simulink model "Simulacao_Exemplo_01"  (R2020a)
settings: Solver=ode45  StartTime=0.0  StopTime=240  FixedStep=0.1  MaxStep=5e-1  RelTol=1e-3  EnableMultiTasking=on
settings Model: Creator=MeneghettiAir  LastModifiedBy=jhona
settings DataIOCC: LimitDataPoints=on  SaveFormat=Array  ReturnWorkspaceOutputs=off
settings OptimizationCC: LifeSpan=inf
settings DebuggingCC: SolverPrmCheckMsg=warning  SFUnexpectedBacktrackingDiag=warning  SFNoUnconditionalDefaultTransitionDiag=warning  SFExecutionAtInitializationDiag=none  ArithmeticOperatorsInVariantConditions=warning
settings HardwareCC: ProdBitPerPointer=32  ProdBitPerSizeT=32  ProdBitPerPtrDiffT=32  ProdLargestAtomicFloat=None  ProdIntDivRoundTo=Undefined  ProdEndianess=Unspecified  ProdWordSize=32  ProdHWDeviceType=32-bit Generic
settings ModelReferenceCC: PropagateSignalLabelsOutOfModel=off
settings SFSimCC: SimUseLocalCustomCode=off  CustomCodeUndefinedFunction=UseInterfaceOnly
settings RTWCC: RTWUseLocalCustomCode=off
settings CodeAppCC: StateflowObjectComments=on
settings GRTTargetCC: TargetLangStandard=C89/C90 (ANSI)
settings ConfigComp: CovMetricSettings=dw  CovHtmlReporting=on  CovSaveCumulativeToWorkspaceVar=on  CovSaveSingleToWorkspaceVar=on  CovExternalEMLEnable=off  CovSFcnEnable=off

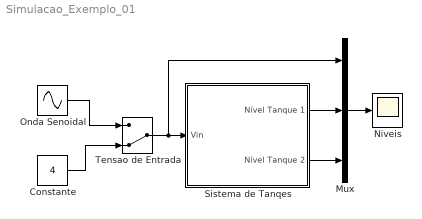
== system Simulacao_Exemplo_01 ==
  Constante : Constant  Value=4  VectorParams1D=off
  Mux : Mux  Inputs=3
  Niveis : Scope
  Onda Senoidal : Sin  Amplitude=2  Bias=2  Frequency=0.2  SampleTime=0
  "Sistema de Tanqes " : Subsystem
  Tensao de Entrada : ManualSwitch  CurrentSetting=0
  wires:
  "Sistema de Tanqes "/1(Nível Tanque 1) -> Mux/2
  "Sistema de Tanqes "/2(Nível Tanque 2) -> Mux/3
  Mux/1 -> Niveis/1
  Tensao de Entrada/1 -> Mux/1, "Sistema de Tanqes "/1(Vin)
  Constante/1 -> Tensao de Entrada/2
  Onda Senoidal/1 -> Tensao de Entrada/1

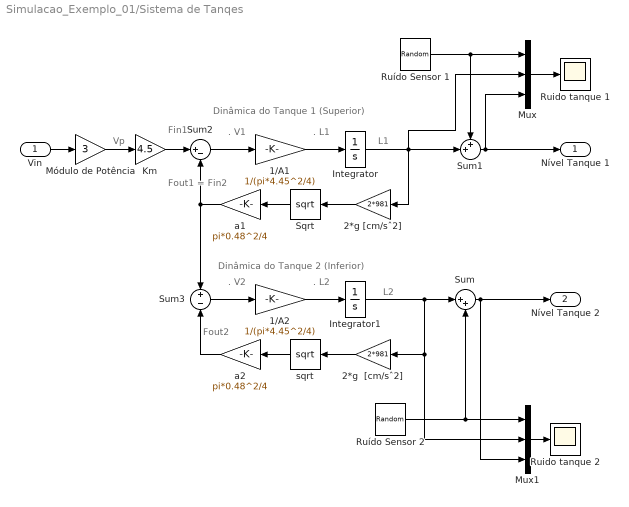
== system Simulacao_Exemplo_01/Sistema de Tanqes  ==
  note: Dinâmica do Tanque 1 (Superior)
  note: L1
  note: Fin1
  note: Fout1
      | =
      | Fin2
  note: .
      | L1
  note: .
      | V1
  note: L2
  note: Fout2
  note: .
      | L2
  note: .
      | V2
  note: Dinâmica do Tanque 2 (Inferior)
  note: Vp
  Vin : Inport
  1/A1 : Gain  Gain=1/(pi*4.45^2/4)
  1/A2 : Gain  Gain=1/(pi*4.45^2/4)
  2*g  [cm/sˆ2] : Gain  Gain=2*981
  2*g [cm/sˆ2] : Gain  Gain=2*981
  Integrator : Integrator  UpperSaturationLimit=35  LowerSaturationLimit=-2
  Integrator1 : Integrator  UpperSaturationLimit=35  LowerSaturationLimit=-2
  Km : Gain  Gain=4.5
  Mux : Mux  Inputs=3
  Mux1 : Mux  Inputs=3
  Módulo de Potência : Gain  Gain=3
  Ruido tanque 1 : Scope
  Ruido tanque 2 : Scope
  Ruído Sensor 1 : UniformRandomNumber  Minimum=-0.5  Maximum=0.5  Seed=round(rand(1)*100)
  Ruído Sensor 2 : UniformRandomNumber  Minimum=-0.5  Maximum=0.5  Seed=round(rand(1)*100)
  Sqrt : Sqrt  SaturateOnIntegerOverflow=on
  Sum : Sum  Inputs=|++
  Sum1 : Sum  Inputs=++|
  Sum2 : Sum  Inputs=|+-
  Sum3 : Sum  Inputs=+-
  a1 : Gain  Gain=pi*0.48^2/4
  a2 : Gain  Gain=pi*0.48^2/4
  sqrt : Sqrt  SaturateOnIntegerOverflow=on
  Nível Tanque 1 : Outport
  Nível Tanque 2 : Outport  Port=2
  wires:
  Vin/1 -> Módulo de Potência/1
  Sum/1 -> Nível Tanque 2/1, Mux1/3
  Mux/1 -> Ruido tanque 1/1
  Mux1/1 -> Ruido tanque 2/1
  Sum1/1 -> Nível Tanque 1/1, Mux/3
  Ruído Sensor 1/1 -> Mux/1, Sum1/1
  Ruído Sensor 2/1 -> Sum/2, Mux1/1
  2*g [cm/sˆ2]/1 -> Sqrt/1
  Sqrt/1 -> a1/1
  Km/1 -> Sum2/1
  a1/1 -> Sum2/2, Sum3/1
  Sum2/1 -> 1/A1/1
  1/A1/1 -> Integrator/1
  2*g  [cm/sˆ2]/1 -> sqrt/1
  sqrt/1 -> a2/1
  Sum3/1 -> 1/A2/1
  1/A2/1 -> Integrator1/1
  a2/1 -> Sum3/2
  Módulo de Potência/1 -> Km/1
  Integrator/1 -> Sum1/2, Mux/2, 2*g [cm/sˆ2]/1
  Integrator1/1 -> Mux1/2, 2*g  [cm/sˆ2]/1, Sum/1
